simulink model "SBR_model"  (R2025a)
settings: Solver=VariableStepAuto  StartTime=0.0  StopTime=10.0  RelTol=1e-3
values from neighbouring files (symbols this model uses):
  beta = 1e-5    (= 1e-05)    [SBR_parameters.m]
  g = 9.81    [SBR_par_separated.m]    (also in SBR_parameters.m; inverse_pendulum.m)
  k = 50    [SBR_parameters.m]
  L = 50e-6    (= 5e-05)    [SBR_par_separated.m]    (also in SBR_parameters.m = 0.01)
  l = 0.25    [SBR_par_separated.m]    (also in SBR_parameters.m = 0.7; inverse_pendulum.m = 0.5)
  m = 0.3    [SBR_par_separated.m]    (also in SBR_parameters.m = 60; inverse_pendulum.m = 1)
  R = 3.5    [SBR_par_separated.m]    (also in SBR_parameters.m = 8)
settings Model: Creator=banom  LastModifiedBy=banom

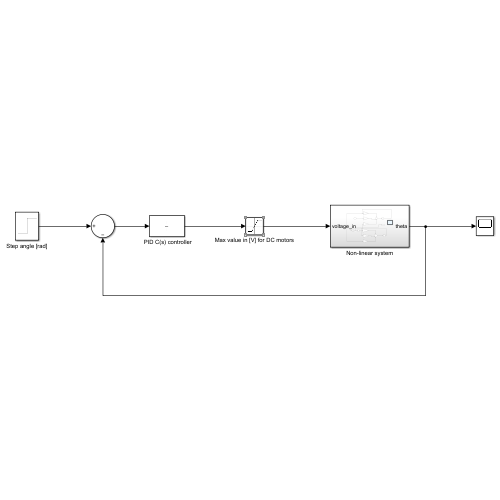
[thumbnail: Simulink's stored preview of the top-level diagram]
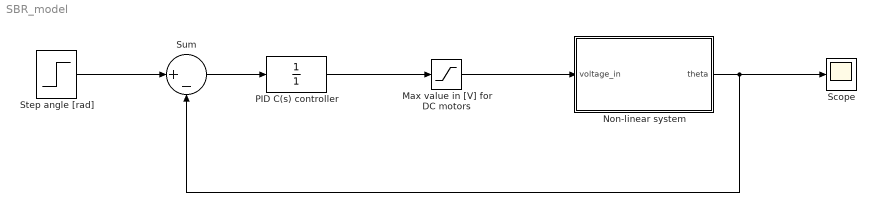
== system SBR_model ==
  " PID C(s) controller" : TransferFcn  Denominator=[1]
  Max value in [V] for DC motors : Saturate
  Non-linear system : Subsystem
  Scope : Scope
  Step angle [rad] : Step  SampleTime=0
  Sum : Sum  Inputs=|+-
  wires:
  Step angle [rad]/1 -> Sum/1
  Sum/1 -> " PID C(s) controller"/1
  " PID C(s) controller"/1 -> Max value in [V] for DC motors/1
  Max value in [V] for DC motors/1 -> Non-linear system/1(voltage_in)
  Non-linear system/1(theta) -> Sum/2, Scope/1

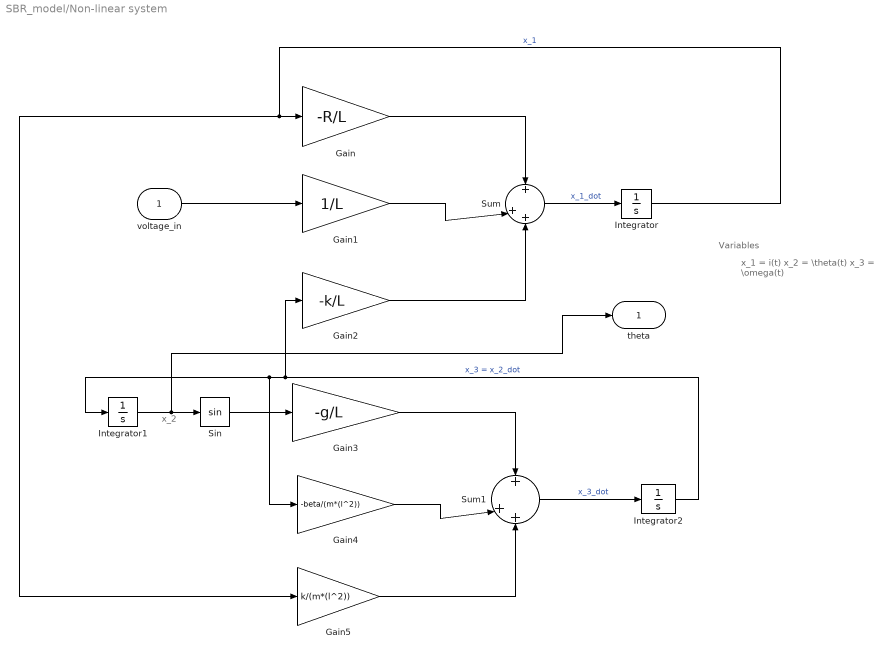
== system SBR_model/Non-linear system ==
  note: x_2
  note: Variables
  note: x_1 = i(t)
      | x_2 = \theta(t)
      | x_3 = \omega(t)
  voltage_in : Inport
  Gain : Gain  Gain=-R/L
  Gain1 : Gain  Gain=1/L
  Gain2 : Gain  Gain=-k/L
  Gain3 : Gain  Gain=-g/L
  Gain4 : Gain  Gain=-beta/(m*(l^2))
  Gain5 : Gain  Gain=k/(m*(l^2))
  Integrator : Integrator
  Integrator1 : Integrator
  Integrator2 : Integrator
  Sin : Trigonometry
  Sum : Sum  Inputs=+|++
  Sum1 : Sum  Inputs=+|++
  theta : Outport
  wires:
  voltage_in/1 -> Gain1/1
  Gain1/1 -> Sum/2
  Gain2/1 -> Sum/3
  Gain/1 -> Sum/1
  Sum/1 -> Integrator/1  "x_1_dot"
  Integrator/1 -> Gain5/1, Gain/1  "x_1"
  Integrator1/1 -> theta/1, Sin/1
  Sin/1 -> Gain3/1
  Gain3/1 -> Sum1/1
  Gain4/1 -> Sum1/2
  Gain5/1 -> Sum1/3
  Sum1/1 -> Integrator2/1  "x_3_dot"
  Integrator2/1 -> Integrator1/1, Gain4/1, Gain2/1  "x_3 = x_2_dot"
